simulink model "dc_dc_fb"  (Simulink 7.9)
settings: Solver=ode23tb  StartTime=0.0  StopTime=0.001  MaxStep=1e-7  RelTol=1e-3  AbsTol=.01
libraries: powerlib x16
settings Model: Creator=lanyi  LastModifiedBy=lanyi
settings OptimizationCC: InlineInvariantSignals=on  InitFltsAndDblsToZero=on
settings DebuggingCC: SaveWithParameterizedLinksMsg=none  SignalResolutionControl=TryResolveAllWithWarning  MultiTaskDSMMsg=warning  MultiTaskCondExecSysMsg=none  FcnCallInpInsideContextMsg=Use local settings  StrictBusMsg=None
settings RTWCC: IncludeERTFirstTime=on
settings GRTTargetCC: TargetFcnLib=ansi_tfl_tmw.mat  CombineOutputUpdateFcns=off  GRTInterface=on

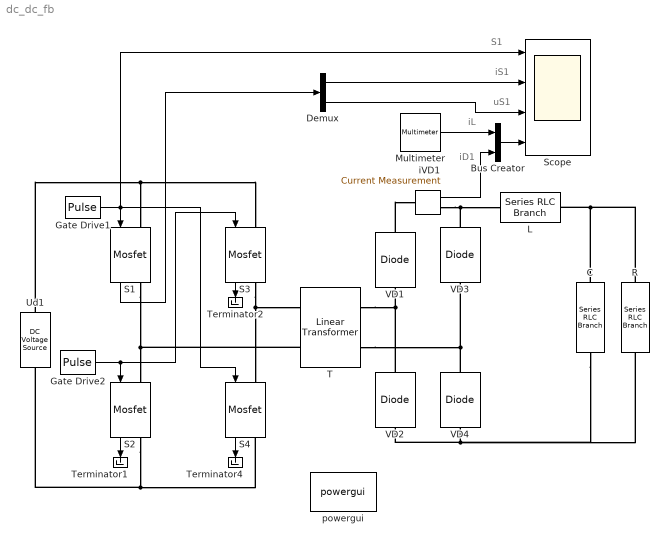
== system dc_dc_fb ==
  note: S1
  note: iL
  note: iS1
  note: uS1
  note: iD1
  Bus Creator : BusCreator  DialogController=Simulink.DDGSource_Bus  Inputs=2
  C : powerlib/Elements/Series RLC Branch  LConnTagsString=__new0  RConnTagsString=__new0  BranchType=C  Resistance=0  Inductance=0  SetiL0=off  InitialCurrent=0  Capacitance=20e-6  Setx0=off  InitialVoltage=0  Measurements=None
  Demux : Demux  Outputs=2
  Gate Drive1 : DiscretePulseGenerator  PulseType=Time based  Period=50e-6  PulseWidth=30
  Gate Drive2 : DiscretePulseGenerator  PulseType=Time based  Period=50e-6  PulseWidth=30  PhaseDelay=25e-6
  L : powerlib/Elements/Series RLC Branch  LConnTagsString=__new0  RConnTagsString=__new0  BranchType=RLC  Resistance=0  Inductance=1e-4  SetiL0=off  InitialCurrent=0  Capacitance=inf  Setx0=off  InitialVoltage=0  Measurements=Branch voltage and current
  Multimeter : powerlib/Measurements/Multimeter  PhasorSimulation=off  OutputType=Complex  sel=5  L=5  Gain=1  yselected={'Ib: L'};  PSBOutputType=1  PSBequivalent=0  AxesSetting=[0,0.1,-100,100]  Display=0  SavedBlockNames=-11
  R : powerlib/Elements/Series RLC Branch  LConnTagsString=__new0  RConnTagsString=__new0  BranchType=R  Resistance=3  Inductance=0  SetiL0=off  InitialCurrent=0  Capacitance=inf  Setx0=off  InitialVoltage=0  Measurements=Branch voltage
  S{1..4} (4 alike) : powerlib/Power Electronics/Mosfet  Ron=0.01  Lon=1e-9  Rd=.01  Vfd=0  IC=0  Rs=30  Cs=1e-8  Measurements=on
  Scope : Scope  NumInputPorts=4
      settings: TimeRange=0.0001  YMin=-0.5~0~0~0  YMax=1.5~25~300~30  SampleTime=1e-7
  T : powerlib/Elements/Linear Transformer  LConnTagsString=a|b  RConnTagsString=A|B  UNITS=pu  NominalPower=[1000 20000 ]  winding1="[200  0.002  0.0002 ]"  winding2="[100  0.002  0.0002 ]"  ThreeWindings=off  winding3=[ 50 0.002 0.002 ]  RmLm=[ 500 20 ]  Measurements=Winding voltages  DataType=off
  Terminator1 : Terminator
  Terminator2 : Terminator
  Terminator4 : Terminator
  Ud1 : powerlib/Electrical Sources/DC Voltage Source  Amplitude=200  Measurements=None
  VD{1..4} (4 alike) : powerlib/Power Electronics/Diode  Ron=0.001  Lon=0  Vf=0.8  IC=0  UseSnubber=off  Rs=100  Cs=1e-9  Measurements=off
  iVD1 : powerlib/Measurements/Current Measurement  PhasorSimulation=off  OutputType=Complex  PSBequivalent=0
  powergui : powerlib/powergui  Priority=1  SimulationMode=Continuous  SolverType=Tustin  SampleTime=50e-6  frequency=60  SPID=off  DisableSnubberDevices=off  DisableRonSwitches=off  DisableVfSwitches=off  SwTol=0  Interpol=off  DisplayEquations=off  FunctionMessages=off  frequencyindice=0  Pbase=100e6  ErrMax=1e-4  Iterations=50  UnitsV=kV  UnitsW=MW  echomessages=off  HookPort=off  EnableUseOfTLC=off  x0status=blocks  RestoreLinks=warning  ResistiveCurrentMeasurement=off  Ylog=off  Xlog=on  ShowGrid=off  save=off  variable=ZData  ZoomFFT=off  StartTime=0.0  cycles=1  DisplayStyle=1  FreqAxis=off  MaxFrequency=1000  frequencyindicesteady=1  display=off  methode=off
  wires:
  Gate Drive1/1 -> S4/1, S1/1, Scope/1
  Multimeter/1 -> Bus Creator/1
  iVD1/1 -> Bus Creator/2
  Gate Drive2/1 -> S2/1, S3/1
  S2/1 -> Terminator1/1
  S4/1 -> Terminator4/1
  S3/1 -> Terminator2/1
  S1/1 -> Demux/1
  Demux/1 -> Scope/2
  Demux/2 -> Scope/3
  Bus Creator/1 -> Scope/4
  connections:
  S2/RConn1 -- S4/RConn1 -- Ud1/LConn1
  S3/RConn1 -- S4/LConn1 -- T/LConn1
  Ud1/RConn1 -- S3/LConn1 -- S1/LConn1
  T/LConn2 -- S2/LConn1 -- S1/RConn1
  C/LConn1 -- R/RConn1 -- VD2/LConn1 -- VD4/LConn1
  T/RConn1 -- VD1/LConn1 -- VD2/RConn1
  R/LConn1 -- L/RConn1 -- C/RConn1
  VD4/RConn1 -- VD3/LConn1 -- T/RConn2
  VD1/RConn1 -- iVD1/LConn1
  iVD1/RConn1 -- L/LConn1 -- VD3/RConn1
